simulink model "Torque_To_Current_Study_ETR07"  (R2017b)
settings: Solver=VariableStepAuto  StartTime=0.0  StopTime=100  RelTol=1e-3
settings Model: Creator=cspt  LastModifiedBy=cspt

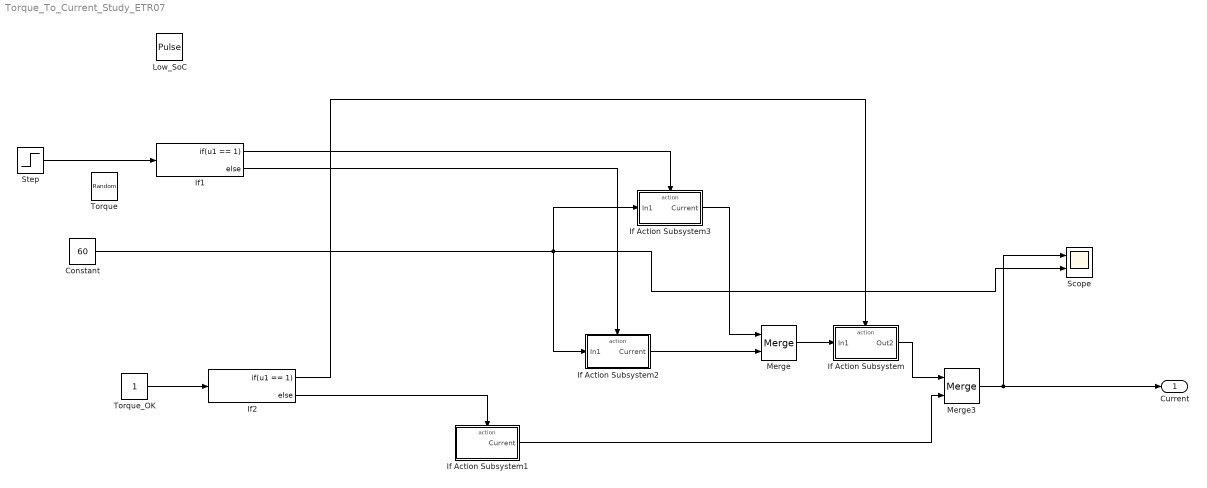
== system Torque_To_Current_Study_ETR07 ==
  Constant : Constant  Value=60
  If Action Subsystem : Subsystem  TreatAsAtomicUnit=on
  If Action Subsystem1 : Subsystem  TreatAsAtomicUnit=on
  If Action Subsystem2 : Subsystem  TreatAsAtomicUnit=on
  If Action Subsystem3 : Subsystem  TreatAsAtomicUnit=on
  If1 : If  IfExpression=u1 == 1
  If2 : If  IfExpression=u1 == 1
  Low_SoC : DiscretePulseGenerator  PulseType=Time based  Period=10  PulseWidth=50
  Merge : Merge
  Merge3 : Merge
  Scope : Scope  NumInputPorts=2
  Step : Step  Time=50  SampleTime=0
  Torque : UniformRandomNumber  Minimum=0  Maximum=140  SampleTime=5
  Torque_OK : Constant
  Current : Outport
  wires:
  If2/1 -> If Action Subsystem/Action
  If2/2 -> If Action Subsystem1/Action
  If Action Subsystem1/1(Current) -> Merge3/2
  Merge3/1 -> Scope/1, Current/1
  Torque_OK/1 -> If2/1
  Step/1 -> If1/1
  If1/2 -> If Action Subsystem2/Action
  If1/1 -> If Action Subsystem3/Action
  If Action Subsystem2/1(Current) -> Merge/2
  If Action Subsystem3/1(Current) -> Merge/1
  Merge/1 -> If Action Subsystem/1(In1)
  If Action Subsystem/1(Out2) -> Merge3/1
  Constant/1 -> If Action Subsystem3/1(In1), If Action Subsystem2/1(In1), Scope/2

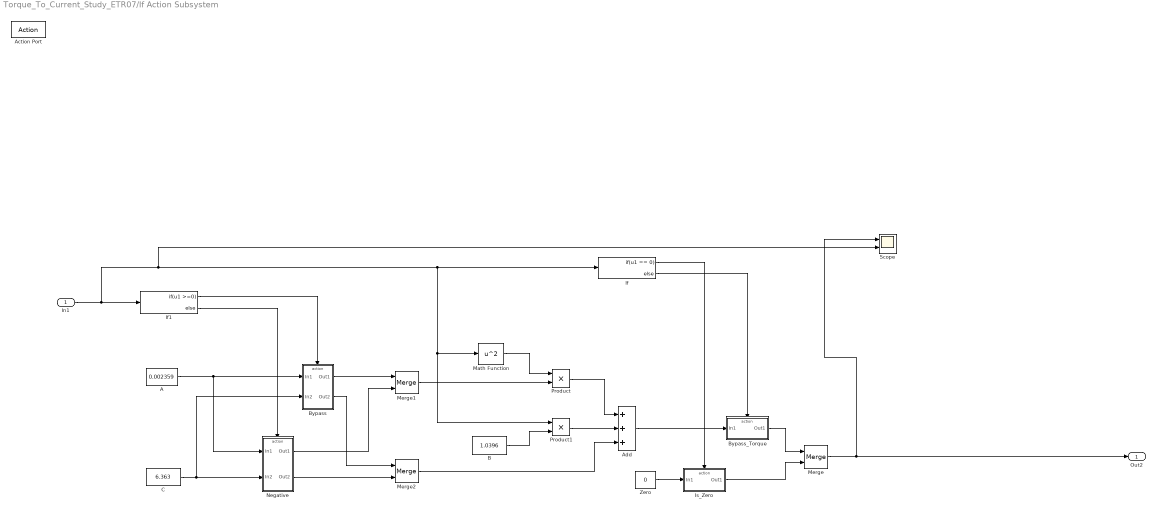
== system Torque_To_Current_Study_ETR07/If Action Subsystem ==
  In1 : Inport
  Action Port : ActionPort  ActionType=then
  A : Constant  Value=0.002359
  Add : Sum  Inputs=+++
  B : Constant  Value=1.0396
  Bypass : Subsystem  TreatAsAtomicUnit=on
  Bypass_Torque : Subsystem  TreatAsAtomicUnit=on
  C : Constant  Value=6.363
  If : If  IfExpression=u1 == 0
  If1 : If  IfExpression=u1 >=0
  Is_Zero : Subsystem  TreatAsAtomicUnit=on
  Math Function : Math  Operator=square  SaturateOnIntegerOverflow=on
  Merge : Merge
  Merge1 : Merge
  Merge2 : Merge
  Negative : Subsystem  TreatAsAtomicUnit=on
  Product : Product
  Product1 : Product
  Scope : Scope  NumInputPorts=2
  Zero : Constant  Value=0
  Out2 : Outport
  wires:
  Is_Zero/1(Out1) -> Merge/2
  Add/1 -> Bypass_Torque/1(In1)
  Bypass/2(Out2) -> Merge2/1
  If/2 -> Bypass_Torque/Action
  Merge1/1 -> Product/2
  B/1 -> Product1/2
  Merge2/1 -> Add/3
  C/1 -> Negative/2(In2), Bypass/2(In2)
  In1/1 -> Scope/2, Product1/1, Math Function/1, If/1, If1/1
  Negative/1(Out1) -> Merge1/2
  Bypass_Torque/1(Out1) -> Merge/1
  Merge/1 -> Out2/1, Scope/1
  A/1 -> Negative/1(In1), Bypass/1(In1)
  Negative/2(Out2) -> Merge2/2
  Product/1 -> Add/1
  Product1/1 -> Add/2
  If/1 -> Is_Zero/Action
  Bypass/1(Out1) -> Merge1/1
  If1/2 -> Negative/Action
  Zero/1 -> Is_Zero/1(In1)
  If1/1 -> Bypass/Action
  Math Function/1 -> Product/1

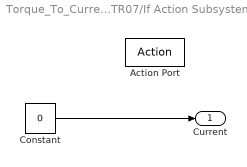
== system Torque_To_Current_Study_ETR07/If Action Subsystem1 ==
  Action Port : ActionPort  ActionType=else
  Constant : Constant  Value=0
  Current : Outport
  wires:
  Constant/1 -> Current/1

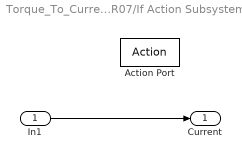
== system Torque_To_Current_Study_ETR07/If Action Subsystem2 ==
  In1 : Inport
  Action Port : ActionPort  ActionType=else
  Current : Outport
  wires:
  In1/1 -> Current/1

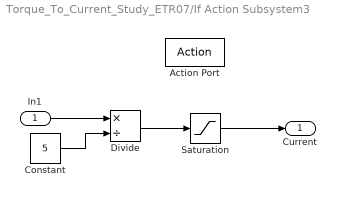
== system Torque_To_Current_Study_ETR07/If Action Subsystem3 ==
  In1 : Inport
  Action Port : ActionPort  ActionType=then
  Constant : Constant  Value=5
  Divide : Product  Inputs=*/
  Saturation : Saturate  UpperLimit=30  LowerLimit=0
  Current : Outport
  wires:
  In1/1 -> Divide/1
  Constant/1 -> Divide/2
  Divide/1 -> Saturation/1
  Saturation/1 -> Current/1

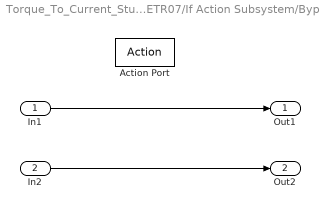
== system Torque_To_Current_Study_ETR07/If Action Subsystem/Bypass ==
  In1 : Inport
  In2 : Inport  Port=2
  Action Port : ActionPort  ActionType=then
  Out1 : Outport
  Out2 : Outport  Port=2
  wires:
  In1/1 -> Out1/1
  In2/1 -> Out2/1

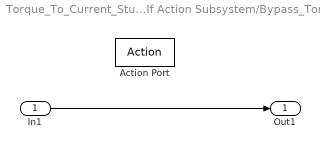
== system Torque_To_Current_Study_ETR07/If Action Subsystem/Bypass_Torque ==
  In1 : Inport
  Action Port : ActionPort  ActionType=else
  Out1 : Outport
  wires:
  In1/1 -> Out1/1

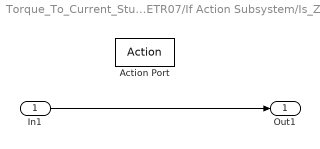
== system Torque_To_Current_Study_ETR07/If Action Subsystem/Is_Zero ==
  In1 : Inport
  Action Port : ActionPort  ActionType=then
  Out1 : Outport
  wires:
  In1/1 -> Out1/1

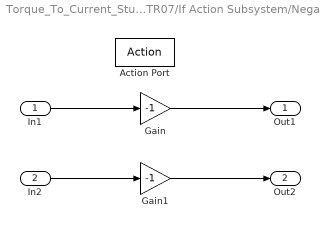
== system Torque_To_Current_Study_ETR07/If Action Subsystem/Negative ==
  In1 : Inport
  In2 : Inport  Port=2
  Action Port : ActionPort  ActionType=else
  Gain : Gain  Gain=-1
  Gain1 : Gain  Gain=-1
  Out1 : Outport
  Out2 : Outport  Port=2
  wires:
  In2/1 -> Gain1/1
  In1/1 -> Gain/1
  Gain/1 -> Out1/1
  Gain1/1 -> Out2/1
